simulink model "mra1gdl"  (Simulink 8.1)
settings: Solver=ode45  StartTime=0.0  StopTime=inf  RelTol=1e-3
undefined symbols (not defined in the file): basec, masac, mra, resortec, RootGround, RootPart
libraries: mblibv1 x14
settings Model: Creator=Liverpool  LastModifiedBy=Daniel
settings DebuggingCC: FcnCallInpInsideContextMsg=EnableAllAsWarning
settings GRTTargetCC: CombineOutputUpdateFcns=on  GRTInterface=off
settings SimMechanicsCC: VisOnUpdateDiagram=on  VisDuringSimulation=on
settings ConfigurationSet: Description=SimMechanics 2G

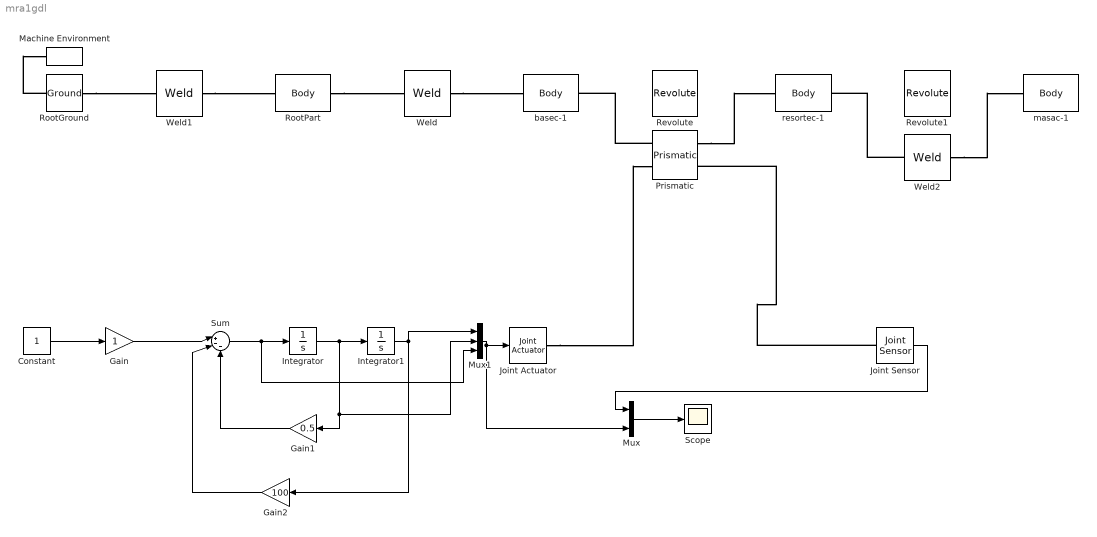
== system mra1gdl ==
  Constant : Constant
  Gain : Gain
  Gain1 : Gain  Gain=0.5
  Gain2 : Gain  Gain=100
  Integrator : Integrator
  Integrator1 : Integrator
  Joint Actuator : mblibv1/Sensors &  Actuators/Joint Actuator  UpdateFromCAD=off  PhysicalDomain=Mechanical  PortType=blob  ActuationStyle=Motion  AngleUnits=deg  ArcVelocityUnits=deg/s  ArcAccelerationUnits=deg/s^2  CoordPositionUnits=m  VelocityUnits=m/s  AccelerationUnits=m/s^2  ForceUnits=mN  TorqueUnits=N*m  ActiveIO=on  Width=3  DialogClass=MechanicalActuatorBlock  Primitive=P1  ReferenceFrame=Absolute (World)
  Joint Sensor : mblibv1/Sensors &  Actuators/Joint Sensor  UpdateFromCAD=off  PhysicalDomain=Mechanical  PortType=blob  Muxed=on  Pose=off  Angle=on  AngleUnits=deg  ArcVelocity=off  ArcVelocityUnits=deg/s  ArcAcceleration=off  ArcAccelerationUnits=deg/s^2  CoordPosition=on  CoordPositionUnits=m  Velocity=off  VelocityUnits=m/s  Acceleration=off  AccelerationUnits=m/s^2  Quaternion=on  QuaternionDT=off  QuaternionDDT=off  QuaternionUnits=off  OutputVector=[1]  ActiveIO=on  Width=1  DialogClass=MechanicalSensorBlock  Primitive=P1  Force=off  ForceUnits=N  Torque=off  TorqueUnits=N-m  ReferenceFrame=Absolute (World)  ReactionSensedSide=Base  ReactionReferenceFrame=Absolute (World)  ReactionForce=off  ReactionForceUnits=N  ReactionMoment=off  ReactionMomentUnits=N-m
  Machine Environment : mblibv1/Bodies/Machine Environment  PortType=env  PhysicalDomain=Mechanical  DialogTemplateClass=MECH.MachineEnvironment  SyncWhenCopied=off  Gravity=[0 -9.81 0]  GravityUnits=m/s^2  GravityAsSignal=off  Dimensionality=Auto-detect  AnalysisType=Forward dynamics  LinearAssemblyTolerance=1e-3  LinearAssemblyToleranceUnits=m  AngularAssemblyTolerance=1e-3  AngularAssemblyToleranceUnits=rad  ConstraintSolverType=Stabilizing  ConstraintRelTolerance=1e-4  ConstraintAbsTolerance=1e-4  UseRobustSingularityHandling=off  RedundancyAnalysisToleranceType=Automatically select tolerance  RedundancyAnalysisTolerance=1e-14  StatePerturbationType=Fixed  PerturbationSize=1e-5  VisualizeMachine=on  BodyVisualizationType=Use model default body geometries  BodyColorSelMode=Use model default  DefaultBodyColor=[1 0 0]
  Mux : Mux  Inputs=2
  Mux1 : Mux  Inputs=3
  Prismatic : mblibv1/Joints/Prismatic  LConnTagsString=__newl0|SA1  RConnTagsString=__newr0|SA1  UpdateFromCAD=off  NumSAPorts=2  CutJoint=off  MarkAsCut=off  Primitives=prismatic  PrimitiveProps=P1$World$[0 1 0]$prismatic  DialogClass=JointBlock  P1Axis=[0 1 0]
  Revolute : mblibv1/Joints/Revolute  LConnTagsString=__newl0  RConnTagsString=__newr0  UpdateFromCAD=on  PMImportedID=basec-1:-:resortec-1  NumSAPorts=0  CutJoint=off  MarkAsCut=off  Primitives=prismatic  PrimitiveProps=R1$WORLD$[0,1,0]$revolute  DialogClass=JointBlock  R1Axis=[0,1,0]
  Revolute1 : mblibv1/Joints/Revolute  LConnTagsString=__newl0  RConnTagsString=__newr0  UpdateFromCAD=on  PMImportedID=masac-1:-:resortec-1  NumSAPorts=0  CutJoint=off  MarkAsCut=off  Primitives=prismatic  PrimitiveProps=R1$WORLD$[0,1,0]$revolute  DialogClass=JointBlock  R1Axis=[0,1,0]
  RootGround : mblibv1/Bodies/Ground  UpdateFromCAD=on  PMImportedID=RootGround  LeftPortType=env  RightPortType=workingframe  PhysicalDomain=Mechanical  DialogClass=GroundBlock  CoordPosition=[-0.00233987,0.00529094,0.1]  CoordPositionUnits=m  StateVectorMgrId=1  MachineId=[2 2]  ShowEnvPort=on
  RootPart : mblibv1/Bodies/Body  LConnTagsString=CS3  RConnTagsString=CS2  UpdateFromCAD=on  PMImportedID=mra/RootPart  DialogClass=MechanicalBodyBlock  Mass=0  MassUnits=kg  InertiaUnits=kg*m^2  Inertia=[0,0,0;0,0,0;0,0,0]  Shape=Cylinder  ShapeDims=[1 1]  ShapeUnits=m  ShapeUse=false  Density=1  DensityUnits=kg/m^3  DensityUse=false  GraphicsMode=MACHINE_DEFAULT  BodyColorSelMode=MACHINE_DEFAULT  BodyColor=[1;0;0]  AttachedToCS=CS1  CG=Right$CG$[-0.00233987 0.00529094 0.1]$WORLD$WORLD$m$[1 0 0;0 1 0;0 0 1]$3x3 Transform$rad$WORLD$false$mra/RootPart::CG(AUTOGEN)  WorkingFrames=Right$CS1$[0 0 0]$WORLD$WORLD$m$[1 0 0;0 1 0;0 0 1]$3x3 Transform$rad$WORLD$false$mra/RootPart::CS1(AUTOGEN)#Right$CS2$[-0.00233987 -0.0340841 0.1]$WORLD$WORLD$m$[1 0 0;0 1 0;0 0 1]$3x3 Transform$rad$WORLD$true$basec-1:-:mra/RootPart::mra/RootPart(AUTOGEN)#Left$CS3$[-0.00233987 0.00529094 0.1]$WORLD$WORLD$m$[1 0 0;0 1 0;0 0 1]$3x3 Transform$rad$WORLD$true$RootGround:-:mra/RootPart::mra/RootPart(AUTOGEN)  CGPos=[-0.00233987 0.00529094 0.1]  CGRot=[1 0 0;0 1 0;0 0 1]  CS0Pos=[]  CS0Rot=[]  CS1Pos=[0 0 0]  CS1Rot=[1 0 0;0 1 0;0 0 1]  CS2Pos=[-0.00233987 -0.0340841 0.1]  CS2Rot=[1 0 0;0 1 0;0 0 1]  CS3Pos=[-0.00233987 0.00529094 0.1]  CS3Rot=[1 0 0;0 1 0;0 0 1]  CS4Pos=[]  CS4Rot=[]  CS5Pos=[]  CS5Rot=[]  CS6Pos=[]  CS6Rot=[]  CS7Pos=[]  CS7Rot=[]  CS8Pos=[]  CS8Rot=[]  CS9Pos=[]  CS9Rot=[]  CS10Pos=[]  CS10Rot=[]  CS11Pos=[]  CS11Rot=[]  CS12Pos=[]  CS12Rot=[]  CS13Pos=[]  CS13Rot=[]  CS14Pos=[]  CS14Rot=[]  CS15Pos=[]  CS15Rot=[]  CS16Pos=[]  CS16Rot=[]  CS17Pos=[]  CS17Rot=[]  CS18Pos=[]  CS18Rot=[]  CS19Pos=[]  CS19Rot=[]  CS20Pos=[]  CS20Rot=[]
  Scope : Scope
  Sum : Sum  Inputs=|+--
  Weld : mblibv1/Joints/Weld  LConnTagsString=__newl0  RConnTagsString=__newr0  UpdateFromCAD=on  PMImportedID=basec-1:-:mra/RootPart  NumSAPorts=0  CutJoint=off  MarkAsCut=off  Primitives=weld  PrimitiveProps=W$WORLD$[0.57735,0.57735,0.57735]$weld  DialogClass=JointBlock  WAxis=[0.57735,0.57735,0.57735]
  Weld1 : mblibv1/Joints/Weld  LConnTagsString=__newl0  RConnTagsString=__newr0  UpdateFromCAD=on  PMImportedID=RootGround:-:mra/RootPart  NumSAPorts=0  CutJoint=off  MarkAsCut=off  Primitives=weld  PrimitiveProps=W$WORLD$[0.57735,0.57735,0.57735]$weld  DialogClass=JointBlock  WAxis=[0.57735,0.57735,0.57735]
  Weld2 : mblibv1/Joints/Weld  LConnTagsString=__newl0  RConnTagsString=__newr0  UpdateFromCAD=on  NumSAPorts=0  CutJoint=off  MarkAsCut=off  Primitives=weld  PrimitiveProps=W$WORLD$[0.57735,0.57735,0.57735]$weld  DialogClass=JointBlock  WAxis=[0.57735,0.57735,0.57735]
  basec-1 : mblibv1/Bodies/Body  LConnTagsString=CS2  RConnTagsString=CS3  UpdateFromCAD=on  PMImportedID=basec-1  DialogClass=MechanicalBodyBlock  Mass=0.0785398  MassUnits=kg  InertiaUnits=kg*m^2  Inertia=[4.97419e-05,0,0;0,9.81748e-05,0;0,0,4.97419e-05]  Shape=Cylinder  ShapeDims=[1 1]  ShapeUnits=m  ShapeUse=false  Density=1  DensityUnits=kg/m^3  DensityUse=false  GraphicsMode=GFXFILE  GraphicsFileName=mra - basec-1.STL  BodyColorSelMode=COLORPALETTE  BodyColor=[0.79216 0.81961 0.93333]  AttachedToCS=CS1  CG=Right$CG$[-0.00233987 -0.0340841 0.1]$WORLD$WORLD$m$[1 0 0;0 1 0;0 0 1]$3x3 Transform$rad$WORLD$false$basec-1::CG(AUTOGEN)  WorkingFrames=Right$CS4$[-0.00233987 -0.0340841 0.1]$WORLD$WORLD$m$[1 0 0;0 1 0;0 0 1]$3x3 Transform$rad$WORLD$false$none#Right$CS1$[-0.00233987 -0.0390841 0.1]$WORLD$WORLD$m$[1 0 0;0 1 0;0 0 1]$3x3 Transform$rad$WORLD$false$basec-1::CS1(AUTOGEN)#Left$CS2$[-0.00233987 -0.0340841 0.1]$WORLD$WORLD$m$[1 0 0;0 1 0;0 0 1]$3x3 Transform$rad$WORLD$true$basec-1:-:mra/RootPart::basec-1(AUTOGEN)#Right$CS3$[-0.00233987 -0.0290841 0.1]$WORLD$WORLD$m$[1 0 0;0 1 0;0 0 1]$3x3 Transform$rad$WORLD$true$basec-1:-:resortec-1::basec-1(AUTOGEN)  CGPos=[-0.00233987 -0.0340841 0.1]  CGRot=[1 0 0;0 1 0;0 0 1]  CS0Pos=[]  CS0Rot=[]  CS1Pos=[-0.00233987 -0.0390841 0.1]  CS1Rot=[1 0 0;0 1 0;0 0 1]  CS2Pos=[-0.00233987 -0.0340841 0.1]  CS2Rot=[1 0 0;0 1 0;0 0 1]  CS3Pos=[-0.00233987 -0.0290841 0.1]  CS3Rot=[1 0 0;0 1 0;0 0 1]  CS4Pos=[-0.00233987 -0.0340841 0.1]  CS4Rot=[1 0 0;0 1 0;0 0 1]  CS5Pos=[]  CS5Rot=[]  CS6Pos=[]  CS6Rot=[]  CS7Pos=[]  CS7Rot=[]  CS8Pos=[]  CS8Rot=[]  CS9Pos=[]  CS9Rot=[]  CS10Pos=[]  CS10Rot=[]  CS11Pos=[]  CS11Rot=[]  CS12Pos=[]  CS12Rot=[]  CS13Pos=[]  CS13Rot=[]  CS14Pos=[]  CS14Rot=[]  CS15Pos=[]  CS15Rot=[]  CS16Pos=[]  CS16Rot=[]  CS17Pos=[]  CS17Rot=[]  CS18Pos=[]  CS18Rot=[]  CS19Pos=[]  CS19Rot=[]  CS20Pos=[]  CS20Rot=[]
  masac-1 : mblibv1/Bodies/Body  LConnTagsString=CS2  UpdateFromCAD=on  PMImportedID=masac-1  DialogClass=MechanicalBodyBlock  Mass=0.0392699  MassUnits=kg  InertiaUnits=kg*m^2  Inertia=[7.44492e-06,0,0;0,1.22718e-05,0;0,0,7.44492e-06]  Shape=Cylinder  ShapeDims=[1 1]  ShapeUnits=m  ShapeUse=false  Density=1  DensityUnits=kg/m^3  DensityUse=false  GraphicsMode=GFXFILE  GraphicsFileName=mra - masac-1.STL  BodyColorSelMode=COLORPALETTE  BodyColor=[0.79216 0.81961 0.93333]  AttachedToCS=CS1  CG=Right$CG$[-0.00233987 0.0809159 0.1]$WORLD$WORLD$m$[0.999375 0 -0.0353606;0 1 0;0.0353606 0 0.999375]$3x3 Transform$rad$WORLD$false$masac-1::CG(AUTOGEN)  WorkingFrames=Left$CS3$[-0.00233987 0.0809159 0.1]$WORLD$WORLD$m$[0.999375 0 -0.0353606;0 1 0;0.0353606 0 0.999375]$3x3 Transform$rad$WORLD$false$none#Left$CS1$[-0.00233987 0.0709159 0.1]$WORLD$WORLD$m$[0.999375 0 -0.0353606;0 1 0;0.0353606 0 0.999375]$3x3 Transform$rad$WORLD$false$masac-1::CS1(AUTOGEN)#Left$CS2$[-0.00233987 0.0709159 0.1]$WORLD$WORLD$m$[1 0 0;0 1 0;0 0 1]$3x3 Transform$rad$WORLD$true$masac-1:-:resortec-1::masac-1(AUTOGEN)  CGPos=[-0.00233987 0.0809159 0.1]  CGRot=[0.999375 0 -0.0353606;0 1 0;0.0353606 0 0.999375]  CS0Pos=[]  CS0Rot=[]  CS1Pos=[-0.00233987 0.0709159 0.1]  CS1Rot=[0.999375 0 -0.0353606;0 1 0;0.0353606 0 0.999375]  CS2Pos=[-0.00233987 0.0709159 0.1]  CS2Rot=[1 0 0;0 1 0;0 0 1]  CS3Pos=[-0.00233987 0.0809159 0.1]  CS3Rot=[0.999375 0 -0.0353606;0 1 0;0.0353606 0 0.999375]  CS4Pos=[]  CS4Rot=[]  CS5Pos=[]  CS5Rot=[]  CS6Pos=[]  CS6Rot=[]  CS7Pos=[]  CS7Rot=[]  CS8Pos=[]  CS8Rot=[]  CS9Pos=[]  CS9Rot=[]  CS10Pos=[]  CS10Rot=[]  CS11Pos=[]  CS11Rot=[]  CS12Pos=[]  CS12Rot=[]  CS13Pos=[]  CS13Rot=[]  CS14Pos=[]  CS14Rot=[]  CS15Pos=[]  CS15Rot=[]  CS16Pos=[]  CS16Rot=[]  CS17Pos=[]  CS17Rot=[]  CS18Pos=[]  CS18Rot=[]  CS19Pos=[]  CS19Rot=[]  CS20Pos=[]  CS20Rot=[]
  resortec-1 : mblibv1/Bodies/Body  LConnTagsString=CS2  RConnTagsString=CS3  UpdateFromCAD=on  PMImportedID=resortec-1  DialogClass=MechanicalBodyBlock  Mass=0.00785398  MassUnits=kg  InertiaUnits=kg*m^2  Inertia=[6.59407e-06,0,0;0,9.81748e-08,0;0,0,6.59407e-06]  Shape=Cylinder  ShapeDims=[1 1]  ShapeUnits=m  ShapeUse=false  Density=1  DensityUnits=kg/m^3  DensityUse=false  GraphicsMode=GFXFILE  GraphicsFileName=mra - resortec-1.STL  BodyColorSelMode=COLORPALETTE  BodyColor=[0.792157;0.819608;0.933333]  AttachedToCS=CS1  CG=Right$CG$[-0.00233987 0.0209159 0.1]$WORLD$WORLD$m$[1 0 0;0 1 0;0 0 1]$3x3 Transform$rad$WORLD$false$resortec-1::CG(AUTOGEN)  WorkingFrames=Right$CS1$[-0.00233987 -0.0290841 0.1]$WORLD$WORLD$m$[1 0 0;0 1 0;0 0 1]$3x3 Transform$rad$WORLD$false$resortec-1::CS1(AUTOGEN)#Left$CS2$[-0.00233987 -0.0290841 0.1]$WORLD$WORLD$m$[1 0 0;0 1 0;0 0 1]$3x3 Transform$rad$WORLD$true$basec-1:-:resortec-1::resortec-1(AUTOGEN)#Right$CS3$[-0.00233987 0.0709159 0.1]$WORLD$WORLD$m$[1 0 0;0 1 0;0 0 1]$3x3 Transform$rad$WORLD$true$masac-1:-:resortec-1::resortec-1(AUTOGEN)  CGPos=[-0.00233987 0.0209159 0.1]  CGRot=[1 0 0;0 1 0;0 0 1]  CS0Pos=[]  CS0Rot=[]  CS1Pos=[-0.00233987 -0.0290841 0.1]  CS1Rot=[1 0 0;0 1 0;0 0 1]  CS2Pos=[-0.00233987 -0.0290841 0.1]  CS2Rot=[1 0 0;0 1 0;0 0 1]  CS3Pos=[-0.00233987 0.0709159 0.1]  CS3Rot=[1 0 0;0 1 0;0 0 1]  CS4Pos=[]  CS4Rot=[]  CS5Pos=[]  CS5Rot=[]  CS6Pos=[]  CS6Rot=[]  CS7Pos=[]  CS7Rot=[]  CS8Pos=[]  CS8Rot=[]  CS9Pos=[]  CS9Rot=[]  CS10Pos=[]  CS10Rot=[]  CS11Pos=[]  CS11Rot=[]  CS12Pos=[]  CS12Rot=[]  CS13Pos=[]  CS13Rot=[]  CS14Pos=[]  CS14Rot=[]  CS15Pos=[]  CS15Rot=[]  CS16Pos=[]  CS16Rot=[]  CS17Pos=[]  CS17Rot=[]  CS18Pos=[]  CS18Rot=[]  CS19Pos=[]  CS19Rot=[]  CS20Pos=[]  CS20Rot=[]
  wires:
  Constant/1 -> Gain/1
  Gain/1 -> Sum/1
  Gain1/1 -> Sum/3
  Gain2/1 -> Sum/2
  Sum/1 -> Integrator/1, Mux1/3
  Integrator/1 -> Integrator1/1, Gain1/1, Mux1/2
  Integrator1/1 -> Gain2/1, Mux1/1
  Mux/1 -> Scope/1
  Joint Sensor/1 -> Mux/1
  Mux1/1 -> Joint Actuator/1, Mux/2
  connections:
  RootPart/RConn1 -- Weld/LConn1
  Weld/RConn1 -- basec-1/LConn1
  RootGround/RConn1 -- Weld1/LConn1
  Weld1/RConn1 -- RootPart/LConn1
  RootGround/LConn1 -- Machine Environment/RConn1
  Weld2/RConn1 -- masac-1/LConn1
  Weld2/LConn1 -- resortec-1/RConn1
  Prismatic/RConn1 -- resortec-1/LConn1
  Prismatic/LConn1 -- basec-1/RConn1
  Joint Sensor/LConn1 -- Prismatic/RConn2
  Joint Actuator/RConn1 -- Prismatic/LConn2
